simulink model "Model_turn"  (R2024a)
settings: Solver=VariableStepAuto  StartTime=0.0  StopTime=100  MaxStep=0.1  RelTol=1e-3
values from neighbouring files (symbols this model uses):
  c_SMA = 837.36    [params.m]
  Fmax_SMA = 10    [params.m]
  h_SMA = .3    (= 0.3)    [params.m]
  k_gn = m*g/0.01    (= 9810)    [contact3D_params.m]
  k_gt = m*g/0.1    (= 981)    [contact3D_params.m]
  m = 10    [contact3D_params.m]
  m_SMA = 0.0025    [params.m]
  max_SMA_Energy_J = 150    [params.m]
  mu_slide = 0.8    [contact3D_params.m]
  mu_stick = 0.9    [contact3D_params.m]
  n_segs = 10    [params.m]
  PWM_max = 0.35    [params.m]
  R_SMA = .08    (= 0.08)    [params.m]
  r_SMA2limb = 0.009    [params.m]
  swing_angle = swing_angles(i)    [params.m]
  T_amb = 23    [params.m]
  V_0 = 7    [params.m]
  v_gn_max = 0.03    [contact3D_params.m]
  v_gt_max = 0.03    [contact3D_params.m]
  vLimit = 0.01    [contact3D_params.m]
undefined symbols (not defined in the file or in its folder): Newton, Raphson, X, Y, Z
libraries: sm_lib x225, nesl_utility x185, simulink x24, simulink_extras x6
(part 12 of 16)

== system Model_turn/LIMB 1: Back LEFT/Limb 1/Limb_Segment5/Limb_Segment_Torques ==
  In1 : Inport
  In2 : Inport  Port=2
  In3 : Inport  Port=3
  In4 : Inport  Port=4
  Constant{,1..3} (4 alike) : Constant  Value=r_SMA2limb
  Gain{,1..3} (4 alike) : Gain  Gain=1/n_segs
  Product{,1..3} (4 alike) : Product
  Simulink-PS Converter : nesl_utility/Simulink-PS Converter  PhysicalDomain=network_engine_domain  SubClassName=ps_input  LeftPortType=input  RightPortType=output  PseudoPeriodic=off  Frequencies=[]  NoiseDistribution=none  NoiseParameters=[]  Unit=1  AffineConversion=off  FilteringAndDerivatives=provide  SimscapeFilterOrder=1  InputFilterTimeConstant=0.001  UdotUserProvided=0
  Simulink-PS Converter1 : nesl_utility/Simulink-PS Converter  PhysicalDomain=network_engine_domain  SubClassName=ps_input  LeftPortType=input  RightPortType=output  PseudoPeriodic=off  Frequencies=[]  NoiseDistribution=none  NoiseParameters=[]  Unit=1  AffineConversion=off  FilteringAndDerivatives=provide  SimscapeFilterOrder=1  InputFilterTimeConstant=0.001  UdotUserProvided=0
  Sum : Sum  Inputs=+-
  Sum1 : Sum  Inputs=+-
  Torque_X : PMIOPort  Side=Right
  Torque_Y : PMIOPort  Port=2  Side=Right
  wires:
  In3/1 -> Gain2/1
  In1/1 -> Gain/1
  In2/1 -> Gain1/1
  Gain1/1 -> Product1/2
  Gain2/1 -> Product2/2
  Gain/1 -> Product/2
  Product/1 -> Sum/1  "SMA_Torque"
  Product2/1 -> Sum1/1  "SMA_Torque"
  Gain3/1 -> Product3/2
  Constant/1 -> Product/1
  Constant1/1 -> Product1/1
  Product1/1 -> Sum/2  "SMA_Torque"
  In4/1 -> Gain3/1
  Constant3/1 -> Product3/1
  Constant2/1 -> Product2/1
  Sum/1 -> Simulink-PS Converter/1
  Product3/1 -> Sum1/2  "SMA_Torque"
  Sum1/1 -> Simulink-PS Converter1/1
  connections:
  Simulink-PS Converter/RConn1 -- Torque_X/RConn1
  Simulink-PS Converter1/RConn1 -- Torque_Y/RConn1

== system Model_turn/LIMB 1: Back LEFT/Limb 1/Limb_Segment6/Limb_Segment_Torques ==
  In1 : Inport
  In2 : Inport  Port=2
  In3 : Inport  Port=3
  In4 : Inport  Port=4
  Constant{,1..3} (4 alike) : Constant  Value=r_SMA2limb
  Gain{,1..3} (4 alike) : Gain  Gain=1/n_segs
  Product{,1..3} (4 alike) : Product
  Simulink-PS Converter : nesl_utility/Simulink-PS Converter  PhysicalDomain=network_engine_domain  SubClassName=ps_input  LeftPortType=input  RightPortType=output  PseudoPeriodic=off  Frequencies=[]  NoiseDistribution=none  NoiseParameters=[]  Unit=1  AffineConversion=off  FilteringAndDerivatives=provide  SimscapeFilterOrder=1  InputFilterTimeConstant=0.001  UdotUserProvided=0
  Simulink-PS Converter1 : nesl_utility/Simulink-PS Converter  PhysicalDomain=network_engine_domain  SubClassName=ps_input  LeftPortType=input  RightPortType=output  PseudoPeriodic=off  Frequencies=[]  NoiseDistribution=none  NoiseParameters=[]  Unit=1  AffineConversion=off  FilteringAndDerivatives=provide  SimscapeFilterOrder=1  InputFilterTimeConstant=0.001  UdotUserProvided=0
  Sum : Sum  Inputs=+-
  Sum1 : Sum  Inputs=+-
  Torque_X : PMIOPort  Side=Right
  Torque_Y : PMIOPort  Port=2  Side=Right
  wires:
  Sum1/1 -> Simulink-PS Converter1/1
  Product3/1 -> Sum1/2  "SMA_Torque"
  Sum/1 -> Simulink-PS Converter/1
  Constant2/1 -> Product2/1
  Constant3/1 -> Product3/1
  In4/1 -> Gain3/1
  Product1/1 -> Sum/2  "SMA_Torque"
  Constant1/1 -> Product1/1
  Constant/1 -> Product/1
  Gain3/1 -> Product3/2
  Product2/1 -> Sum1/1  "SMA_Torque"
  Product/1 -> Sum/1  "SMA_Torque"
  Gain/1 -> Product/2
  Gain2/1 -> Product2/2
  Gain1/1 -> Product1/2
  In2/1 -> Gain1/1
  In1/1 -> Gain/1
  In3/1 -> Gain2/1
  connections:
  Simulink-PS Converter1/RConn1 -- Torque_Y/RConn1
  Simulink-PS Converter/RConn1 -- Torque_X/RConn1

== system Model_turn/LIMB 1: Back LEFT/Limb 1/Limb_Segment7/Limb_Segment_Torques ==
  In1 : Inport
  In2 : Inport  Port=2
  In3 : Inport  Port=3
  In4 : Inport  Port=4
  Constant{,1..3} (4 alike) : Constant  Value=r_SMA2limb
  Gain{,1..3} (4 alike) : Gain  Gain=1/n_segs
  Product{,1..3} (4 alike) : Product
  Simulink-PS Converter : nesl_utility/Simulink-PS Converter  PhysicalDomain=network_engine_domain  SubClassName=ps_input  LeftPortType=input  RightPortType=output  PseudoPeriodic=off  Frequencies=[]  NoiseDistribution=none  NoiseParameters=[]  Unit=1  AffineConversion=off  FilteringAndDerivatives=provide  SimscapeFilterOrder=1  InputFilterTimeConstant=0.001  UdotUserProvided=0
  Simulink-PS Converter1 : nesl_utility/Simulink-PS Converter  PhysicalDomain=network_engine_domain  SubClassName=ps_input  LeftPortType=input  RightPortType=output  PseudoPeriodic=off  Frequencies=[]  NoiseDistribution=none  NoiseParameters=[]  Unit=1  AffineConversion=off  FilteringAndDerivatives=provide  SimscapeFilterOrder=1  InputFilterTimeConstant=0.001  UdotUserProvided=0
  Sum : Sum  Inputs=+-
  Sum1 : Sum  Inputs=+-
  Torque_X : PMIOPort  Side=Right
  Torque_Y : PMIOPort  Port=2  Side=Right
  wires:
  In3/1 -> Gain2/1
  In1/1 -> Gain/1
  In2/1 -> Gain1/1
  Gain1/1 -> Product1/2
  Gain2/1 -> Product2/2
  Gain/1 -> Product/2
  Product/1 -> Sum/1  "SMA_Torque"
  Product2/1 -> Sum1/1  "SMA_Torque"
  Gain3/1 -> Product3/2
  Constant/1 -> Product/1
  Constant1/1 -> Product1/1
  Product1/1 -> Sum/2  "SMA_Torque"
  In4/1 -> Gain3/1
  Constant3/1 -> Product3/1
  Constant2/1 -> Product2/1
  Sum/1 -> Simulink-PS Converter/1
  Product3/1 -> Sum1/2  "SMA_Torque"
  Sum1/1 -> Simulink-PS Converter1/1
  connections:
  Simulink-PS Converter/RConn1 -- Torque_X/RConn1
  Simulink-PS Converter1/RConn1 -- Torque_Y/RConn1

== system Model_turn/LIMB 1: Back LEFT/Limb 1/Limb_Segment8/Limb_Segment_Torques ==
  In1 : Inport
  In2 : Inport  Port=2
  In3 : Inport  Port=3
  In4 : Inport  Port=4
  Constant{,1..3} (4 alike) : Constant  Value=r_SMA2limb
  Gain{,1..3} (4 alike) : Gain  Gain=1/n_segs
  Product{,1..3} (4 alike) : Product
  Simulink-PS Converter : nesl_utility/Simulink-PS Converter  PhysicalDomain=network_engine_domain  SubClassName=ps_input  LeftPortType=input  RightPortType=output  PseudoPeriodic=off  Frequencies=[]  NoiseDistribution=none  NoiseParameters=[]  Unit=1  AffineConversion=off  FilteringAndDerivatives=provide  SimscapeFilterOrder=1  InputFilterTimeConstant=0.001  UdotUserProvided=0
  Simulink-PS Converter1 : nesl_utility/Simulink-PS Converter  PhysicalDomain=network_engine_domain  SubClassName=ps_input  LeftPortType=input  RightPortType=output  PseudoPeriodic=off  Frequencies=[]  NoiseDistribution=none  NoiseParameters=[]  Unit=1  AffineConversion=off  FilteringAndDerivatives=provide  SimscapeFilterOrder=1  InputFilterTimeConstant=0.001  UdotUserProvided=0
  Sum : Sum  Inputs=+-
  Sum1 : Sum  Inputs=+-
  Torque_X : PMIOPort  Side=Right
  Torque_Y : PMIOPort  Port=2  Side=Right
  wires:
  Sum1/1 -> Simulink-PS Converter1/1
  Product3/1 -> Sum1/2  "SMA_Torque"
  Sum/1 -> Simulink-PS Converter/1
  Constant2/1 -> Product2/1
  Constant3/1 -> Product3/1
  In4/1 -> Gain3/1
  Product1/1 -> Sum/2  "SMA_Torque"
  Constant1/1 -> Product1/1
  Constant/1 -> Product/1
  Gain3/1 -> Product3/2
  Product2/1 -> Sum1/1  "SMA_Torque"
  Product/1 -> Sum/1  "SMA_Torque"
  Gain/1 -> Product/2
  Gain2/1 -> Product2/2
  Gain1/1 -> Product1/2
  In2/1 -> Gain1/1
  In1/1 -> Gain/1
  In3/1 -> Gain2/1
  connections:
  Simulink-PS Converter1/RConn1 -- Torque_Y/RConn1
  Simulink-PS Converter/RConn1 -- Torque_X/RConn1

== system Model_turn/LIMB 1: Back LEFT/Limb 1/Limb_Segment9/Limb_Segment_Torques ==
  In1 : Inport
  In2 : Inport  Port=2
  In3 : Inport  Port=3
  In4 : Inport  Port=4
  Constant{,1..3} (4 alike) : Constant  Value=r_SMA2limb
  Gain{,1..3} (4 alike) : Gain  Gain=1/n_segs
  Product{,1..3} (4 alike) : Product
  Simulink-PS Converter : nesl_utility/Simulink-PS Converter  PhysicalDomain=network_engine_domain  SubClassName=ps_input  LeftPortType=input  RightPortType=output  PseudoPeriodic=off  Frequencies=[]  NoiseDistribution=none  NoiseParameters=[]  Unit=1  AffineConversion=off  FilteringAndDerivatives=provide  SimscapeFilterOrder=1  InputFilterTimeConstant=0.001  UdotUserProvided=0
  Simulink-PS Converter1 : nesl_utility/Simulink-PS Converter  PhysicalDomain=network_engine_domain  SubClassName=ps_input  LeftPortType=input  RightPortType=output  PseudoPeriodic=off  Frequencies=[]  NoiseDistribution=none  NoiseParameters=[]  Unit=1  AffineConversion=off  FilteringAndDerivatives=provide  SimscapeFilterOrder=1  InputFilterTimeConstant=0.001  UdotUserProvided=0
  Sum : Sum  Inputs=+-
  Sum1 : Sum  Inputs=+-
  Torque_X : PMIOPort  Side=Right
  Torque_Y : PMIOPort  Port=2  Side=Right
  wires:
  In3/1 -> Gain2/1
  In1/1 -> Gain/1
  In2/1 -> Gain1/1
  Gain1/1 -> Product1/2
  Gain2/1 -> Product2/2
  Gain/1 -> Product/2
  Product/1 -> Sum/1  "SMA_Torque"
  Product2/1 -> Sum1/1  "SMA_Torque"
  Gain3/1 -> Product3/2
  Constant/1 -> Product/1
  Constant1/1 -> Product1/1
  Product1/1 -> Sum/2  "SMA_Torque"
  In4/1 -> Gain3/1
  Constant3/1 -> Product3/1
  Constant2/1 -> Product2/1
  Sum/1 -> Simulink-PS Converter/1
  Product3/1 -> Sum1/2  "SMA_Torque"
  Sum1/1 -> Simulink-PS Converter1/1
  connections:
  Simulink-PS Converter/RConn1 -- Torque_X/RConn1
  Simulink-PS Converter1/RConn1 -- Torque_Y/RConn1

== system Model_turn/LIMB 1: Back LEFT/Limb 1/Right Ball Contact/3D Contact ==
  RefPt [m m m] : Inport
  nVec [m m m] : Inport  Port=2
  pVec [m m m] : Inport  Port=3
  vVec [m/s m/s m/s] : Inport  Port=4
  Contact! : EnablePort  StatesWhenEnabling=reset
  Friction Switch : Subsystem
  Kinetic Friction Model : Subsystem
  Logical Operator : Logic  Operator=NOT  AllPortsSameDT=off  OutDataTypeStr=boolean
  Static Friction Model : Subsystem
  Sum : Sum
  Sum1 : Sum
  FnVec [N N N] : Outport  OutputWhenDisabled=reset  InitialOutput=[0 0 0]
      settings: AttributesFormatString=when disabled: %<OutputWhenDisabled>
  FtVec [N N N] : Outport  Port=2  OutputWhenDisabled=reset  InitialOutput=[0 0 0]
      settings: AttributesFormatString=when disabled: %<OutputWhenDisabled>
  wires:
  pVec [m m m]/1 -> Static Friction Model/1(pos [m]), Kinetic Friction Model/2(pos [m m m])
  vVec [m/s m/s m/s]/1 -> Kinetic Friction Model/1(vel [m/s m/s m/s]), Static Friction Model/2(vel [m/s m/s m/s])
  Kinetic Friction Model/2(posFP [m m m]) -> Static Friction Model/4(posFP [m])
  Friction Switch/1(Stiction) -> Static Friction Model/Enable, Logical Operator/1
  Logical Operator/1 -> Kinetic Friction Model/Enable
  nVec [m m m]/1 -> Kinetic Friction Model/4(nVec [m m m])
  Kinetic Friction Model/4(Stiction!) -> Friction Switch/2(Stick!)
  Static Friction Model/1(F_n Stick [N N N]) -> Sum1/1
  Kinetic Friction Model/6(F_n Slide [N N N]) -> Sum1/2
  Kinetic Friction Model/5(F_t Slide [N N N]) -> Sum/2
  Static Friction Model/2(F_t Stick [N N N]) -> Sum/1
  Sum1/1 -> FnVec [N N N]/1  "F_nVec"
  Sum/1 -> FtVec [N N N]/1  "F_tVec"
  Static Friction Model/3(Sliding!) -> Friction Switch/1(Slide!)
  RefPt [m m m]/1 -> Kinetic Friction Model/3(RefPt [m m m])
  Kinetic Friction Model/3(nVec FP [m m m]) -> Static Friction Model/5(nVecFP [m m m])
  Kinetic Friction Model/1(RefPtFP [m m m]) -> Static Friction Model/3(RefPtFP [m m m])

== system Model_turn/LIMB 1: Back RIGHT/Limb 1/Limb_Segment/Limb_Segment_Torques ==
  In1 : Inport
  In2 : Inport  Port=2
  In3 : Inport  Port=3
  In4 : Inport  Port=4
  Constant{,1..3} (4 alike) : Constant  Value=r_SMA2limb
  Gain{,1..3} (4 alike) : Gain  Gain=1/n_segs
  Product{,1..3} (4 alike) : Product
  Simulink-PS Converter : nesl_utility/Simulink-PS Converter  PhysicalDomain=network_engine_domain  SubClassName=ps_input  LeftPortType=input  RightPortType=output  PseudoPeriodic=off  Frequencies=[]  NoiseDistribution=none  NoiseParameters=[]  Unit=1  AffineConversion=off  FilteringAndDerivatives=provide  SimscapeFilterOrder=1  InputFilterTimeConstant=0.001  UdotUserProvided=0
  Simulink-PS Converter1 : nesl_utility/Simulink-PS Converter  PhysicalDomain=network_engine_domain  SubClassName=ps_input  LeftPortType=input  RightPortType=output  PseudoPeriodic=off  Frequencies=[]  NoiseDistribution=none  NoiseParameters=[]  Unit=1  AffineConversion=off  FilteringAndDerivatives=provide  SimscapeFilterOrder=1  InputFilterTimeConstant=0.001  UdotUserProvided=0
  Sum : Sum  Inputs=+-
  Sum1 : Sum  Inputs=+-
  Torque_X : PMIOPort  Side=Right
  Torque_Y : PMIOPort  Port=2  Side=Right
  wires:
  Sum1/1 -> Simulink-PS Converter1/1
  Product3/1 -> Sum1/2  "SMA_Torque"
  Sum/1 -> Simulink-PS Converter/1
  Constant2/1 -> Product2/1
  Constant3/1 -> Product3/1
  In4/1 -> Gain3/1
  Product1/1 -> Sum/2  "SMA_Torque"
  Constant1/1 -> Product1/1
  Constant/1 -> Product/1
  Gain3/1 -> Product3/2
  Product2/1 -> Sum1/1  "SMA_Torque"
  Product/1 -> Sum/1  "SMA_Torque"
  Gain/1 -> Product/2
  Gain2/1 -> Product2/2
  Gain1/1 -> Product1/2
  In2/1 -> Gain1/1
  In1/1 -> Gain/1
  In3/1 -> Gain2/1
  connections:
  Simulink-PS Converter1/RConn1 -- Torque_Y/RConn1
  Simulink-PS Converter/RConn1 -- Torque_X/RConn1

== system Model_turn/LIMB 1: Back RIGHT/Limb 1/Limb_Segment1/Limb_Segment_Torques ==
  In1 : Inport
  In2 : Inport  Port=2
  In3 : Inport  Port=3
  In4 : Inport  Port=4
  Constant{,1..3} (4 alike) : Constant  Value=r_SMA2limb
  Gain{,1..3} (4 alike) : Gain  Gain=1/n_segs
  Product{,1..3} (4 alike) : Product
  Simulink-PS Converter : nesl_utility/Simulink-PS Converter  PhysicalDomain=network_engine_domain  SubClassName=ps_input  LeftPortType=input  RightPortType=output  PseudoPeriodic=off  Frequencies=[]  NoiseDistribution=none  NoiseParameters=[]  Unit=1  AffineConversion=off  FilteringAndDerivatives=provide  SimscapeFilterOrder=1  InputFilterTimeConstant=0.001  UdotUserProvided=0
  Simulink-PS Converter1 : nesl_utility/Simulink-PS Converter  PhysicalDomain=network_engine_domain  SubClassName=ps_input  LeftPortType=input  RightPortType=output  PseudoPeriodic=off  Frequencies=[]  NoiseDistribution=none  NoiseParameters=[]  Unit=1  AffineConversion=off  FilteringAndDerivatives=provide  SimscapeFilterOrder=1  InputFilterTimeConstant=0.001  UdotUserProvided=0
  Sum : Sum  Inputs=+-
  Sum1 : Sum  Inputs=+-
  Torque_X : PMIOPort  Side=Right
  Torque_Y : PMIOPort  Port=2  Side=Right
  wires:
  In3/1 -> Gain2/1
  In1/1 -> Gain/1
  In2/1 -> Gain1/1
  Gain1/1 -> Product1/2
  Gain2/1 -> Product2/2
  Gain/1 -> Product/2
  Product/1 -> Sum/1  "SMA_Torque"
  Product2/1 -> Sum1/1  "SMA_Torque"
  Gain3/1 -> Product3/2
  Constant/1 -> Product/1
  Constant1/1 -> Product1/1
  Product1/1 -> Sum/2  "SMA_Torque"
  In4/1 -> Gain3/1
  Constant3/1 -> Product3/1
  Constant2/1 -> Product2/1
  Sum/1 -> Simulink-PS Converter/1
  Product3/1 -> Sum1/2  "SMA_Torque"
  Sum1/1 -> Simulink-PS Converter1/1
  connections:
  Simulink-PS Converter/RConn1 -- Torque_X/RConn1
  Simulink-PS Converter1/RConn1 -- Torque_Y/RConn1

== system Model_turn/LIMB 1: Back RIGHT/Limb 1/Limb_Segment2/Limb_Segment_Torques ==
  In1 : Inport
  In2 : Inport  Port=2
  In3 : Inport  Port=3
  In4 : Inport  Port=4
  Constant{,1..3} (4 alike) : Constant  Value=r_SMA2limb
  Gain{,1..3} (4 alike) : Gain  Gain=1/n_segs
  Product{,1..3} (4 alike) : Product
  Simulink-PS Converter : nesl_utility/Simulink-PS Converter  PhysicalDomain=network_engine_domain  SubClassName=ps_input  LeftPortType=input  RightPortType=output  PseudoPeriodic=off  Frequencies=[]  NoiseDistribution=none  NoiseParameters=[]  Unit=1  AffineConversion=off  FilteringAndDerivatives=provide  SimscapeFilterOrder=1  InputFilterTimeConstant=0.001  UdotUserProvided=0
  Simulink-PS Converter1 : nesl_utility/Simulink-PS Converter  PhysicalDomain=network_engine_domain  SubClassName=ps_input  LeftPortType=input  RightPortType=output  PseudoPeriodic=off  Frequencies=[]  NoiseDistribution=none  NoiseParameters=[]  Unit=1  AffineConversion=off  FilteringAndDerivatives=provide  SimscapeFilterOrder=1  InputFilterTimeConstant=0.001  UdotUserProvided=0
  Sum : Sum  Inputs=+-
  Sum1 : Sum  Inputs=+-
  Torque_X : PMIOPort  Side=Right
  Torque_Y : PMIOPort  Port=2  Side=Right
  wires:
  Sum1/1 -> Simulink-PS Converter1/1
  Product3/1 -> Sum1/2  "SMA_Torque"
  Sum/1 -> Simulink-PS Converter/1
  Constant2/1 -> Product2/1
  Constant3/1 -> Product3/1
  In4/1 -> Gain3/1
  Product1/1 -> Sum/2  "SMA_Torque"
  Constant1/1 -> Product1/1
  Constant/1 -> Product/1
  Gain3/1 -> Product3/2
  Product2/1 -> Sum1/1  "SMA_Torque"
  Product/1 -> Sum/1  "SMA_Torque"
  Gain/1 -> Product/2
  Gain2/1 -> Product2/2
  Gain1/1 -> Product1/2
  In2/1 -> Gain1/1
  In1/1 -> Gain/1
  In3/1 -> Gain2/1
  connections:
  Simulink-PS Converter1/RConn1 -- Torque_Y/RConn1
  Simulink-PS Converter/RConn1 -- Torque_X/RConn1

== system Model_turn/LIMB 1: Back RIGHT/Limb 1/Limb_Segment3/Limb_Segment_Torques ==
  In1 : Inport
  In2 : Inport  Port=2
  In3 : Inport  Port=3
  In4 : Inport  Port=4
  Constant{,1..3} (4 alike) : Constant  Value=r_SMA2limb
  Gain{,1..3} (4 alike) : Gain  Gain=1/n_segs
  Product{,1..3} (4 alike) : Product
  Simulink-PS Converter : nesl_utility/Simulink-PS Converter  PhysicalDomain=network_engine_domain  SubClassName=ps_input  LeftPortType=input  RightPortType=output  PseudoPeriodic=off  Frequencies=[]  NoiseDistribution=none  NoiseParameters=[]  Unit=1  AffineConversion=off  FilteringAndDerivatives=provide  SimscapeFilterOrder=1  InputFilterTimeConstant=0.001  UdotUserProvided=0
  Simulink-PS Converter1 : nesl_utility/Simulink-PS Converter  PhysicalDomain=network_engine_domain  SubClassName=ps_input  LeftPortType=input  RightPortType=output  PseudoPeriodic=off  Frequencies=[]  NoiseDistribution=none  NoiseParameters=[]  Unit=1  AffineConversion=off  FilteringAndDerivatives=provide  SimscapeFilterOrder=1  InputFilterTimeConstant=0.001  UdotUserProvided=0
  Sum : Sum  Inputs=+-
  Sum1 : Sum  Inputs=+-
  Torque_X : PMIOPort  Side=Right
  Torque_Y : PMIOPort  Port=2  Side=Right
  wires:
  In3/1 -> Gain2/1
  In1/1 -> Gain/1
  In2/1 -> Gain1/1
  Gain1/1 -> Product1/2
  Gain2/1 -> Product2/2
  Gain/1 -> Product/2
  Product/1 -> Sum/1  "SMA_Torque"
  Product2/1 -> Sum1/1  "SMA_Torque"
  Gain3/1 -> Product3/2
  Constant/1 -> Product/1
  Constant1/1 -> Product1/1
  Product1/1 -> Sum/2  "SMA_Torque"
  In4/1 -> Gain3/1
  Constant3/1 -> Product3/1
  Constant2/1 -> Product2/1
  Sum/1 -> Simulink-PS Converter/1
  Product3/1 -> Sum1/2  "SMA_Torque"
  Sum1/1 -> Simulink-PS Converter1/1
  connections:
  Simulink-PS Converter/RConn1 -- Torque_X/RConn1
  Simulink-PS Converter1/RConn1 -- Torque_Y/RConn1

== system Model_turn/LIMB 1: Back RIGHT/Limb 1/Limb_Segment4/Limb_Segment_Torques ==
  In1 : Inport
  In2 : Inport  Port=2
  In3 : Inport  Port=3
  In4 : Inport  Port=4
  Constant{,1..3} (4 alike) : Constant  Value=r_SMA2limb
  Gain{,1..3} (4 alike) : Gain  Gain=1/n_segs
  Product{,1..3} (4 alike) : Product
  Simulink-PS Converter : nesl_utility/Simulink-PS Converter  PhysicalDomain=network_engine_domain  SubClassName=ps_input  LeftPortType=input  RightPortType=output  PseudoPeriodic=off  Frequencies=[]  NoiseDistribution=none  NoiseParameters=[]  Unit=1  AffineConversion=off  FilteringAndDerivatives=provide  SimscapeFilterOrder=1  InputFilterTimeConstant=0.001  UdotUserProvided=0
  Simulink-PS Converter1 : nesl_utility/Simulink-PS Converter  PhysicalDomain=network_engine_domain  SubClassName=ps_input  LeftPortType=input  RightPortType=output  PseudoPeriodic=off  Frequencies=[]  NoiseDistribution=none  NoiseParameters=[]  Unit=1  AffineConversion=off  FilteringAndDerivatives=provide  SimscapeFilterOrder=1  InputFilterTimeConstant=0.001  UdotUserProvided=0
  Sum : Sum  Inputs=+-
  Sum1 : Sum  Inputs=+-
  Torque_X : PMIOPort  Side=Right
  Torque_Y : PMIOPort  Port=2  Side=Right
  wires:
  Sum1/1 -> Simulink-PS Converter1/1
  Product3/1 -> Sum1/2  "SMA_Torque"
  Sum/1 -> Simulink-PS Converter/1
  Constant2/1 -> Product2/1
  Constant3/1 -> Product3/1
  In4/1 -> Gain3/1
  Product1/1 -> Sum/2  "SMA_Torque"
  Constant1/1 -> Product1/1
  Constant/1 -> Product/1
  Gain3/1 -> Product3/2
  Product2/1 -> Sum1/1  "SMA_Torque"
  Product/1 -> Sum/1  "SMA_Torque"
  Gain/1 -> Product/2
  Gain2/1 -> Product2/2
  Gain1/1 -> Product1/2
  In2/1 -> Gain1/1
  In1/1 -> Gain/1
  In3/1 -> Gain2/1
  connections:
  Simulink-PS Converter1/RConn1 -- Torque_Y/RConn1
  Simulink-PS Converter/RConn1 -- Torque_X/RConn1

== system Model_turn/LIMB 1: Back RIGHT/Limb 1/Limb_Segment5/Limb_Segment_Torques ==
  In1 : Inport
  In2 : Inport  Port=2
  In3 : Inport  Port=3
  In4 : Inport  Port=4
  Constant{,1..3} (4 alike) : Constant  Value=r_SMA2limb
  Gain{,1..3} (4 alike) : Gain  Gain=1/n_segs
  Product{,1..3} (4 alike) : Product
  Simulink-PS Converter : nesl_utility/Simulink-PS Converter  PhysicalDomain=network_engine_domain  SubClassName=ps_input  LeftPortType=input  RightPortType=output  PseudoPeriodic=off  Frequencies=[]  NoiseDistribution=none  NoiseParameters=[]  Unit=1  AffineConversion=off  FilteringAndDerivatives=provide  SimscapeFilterOrder=1  InputFilterTimeConstant=0.001  UdotUserProvided=0
  Simulink-PS Converter1 : nesl_utility/Simulink-PS Converter  PhysicalDomain=network_engine_domain  SubClassName=ps_input  LeftPortType=input  RightPortType=output  PseudoPeriodic=off  Frequencies=[]  NoiseDistribution=none  NoiseParameters=[]  Unit=1  AffineConversion=off  FilteringAndDerivatives=provide  SimscapeFilterOrder=1  InputFilterTimeConstant=0.001  UdotUserProvided=0
  Sum : Sum  Inputs=+-
  Sum1 : Sum  Inputs=+-
  Torque_X : PMIOPort  Side=Right
  Torque_Y : PMIOPort  Port=2  Side=Right
  wires:
  Sum1/1 -> Simulink-PS Converter1/1
  Product3/1 -> Sum1/2  "SMA_Torque"
  Sum/1 -> Simulink-PS Converter/1
  Constant2/1 -> Product2/1
  Constant3/1 -> Product3/1
  In4/1 -> Gain3/1
  Product1/1 -> Sum/2  "SMA_Torque"
  Constant1/1 -> Product1/1
  Constant/1 -> Product/1
  Gain3/1 -> Product3/2
  Product2/1 -> Sum1/1  "SMA_Torque"
  Product/1 -> Sum/1  "SMA_Torque"
  Gain/1 -> Product/2
  Gain2/1 -> Product2/2
  Gain1/1 -> Product1/2
  In2/1 -> Gain1/1
  In1/1 -> Gain/1
  In3/1 -> Gain2/1
  connections:
  Simulink-PS Converter1/RConn1 -- Torque_Y/RConn1
  Simulink-PS Converter/RConn1 -- Torque_X/RConn1

== system Model_turn/LIMB 1: Back RIGHT/Limb 1/Limb_Segment6/Limb_Segment_Torques ==
  In1 : Inport
  In2 : Inport  Port=2
  In3 : Inport  Port=3
  In4 : Inport  Port=4
  Constant{,1..3} (4 alike) : Constant  Value=r_SMA2limb
  Gain{,1..3} (4 alike) : Gain  Gain=1/n_segs
  Product{,1..3} (4 alike) : Product
  Simulink-PS Converter : nesl_utility/Simulink-PS Converter  PhysicalDomain=network_engine_domain  SubClassName=ps_input  LeftPortType=input  RightPortType=output  PseudoPeriodic=off  Frequencies=[]  NoiseDistribution=none  NoiseParameters=[]  Unit=1  AffineConversion=off  FilteringAndDerivatives=provide  SimscapeFilterOrder=1  InputFilterTimeConstant=0.001  UdotUserProvided=0
  Simulink-PS Converter1 : nesl_utility/Simulink-PS Converter  PhysicalDomain=network_engine_domain  SubClassName=ps_input  LeftPortType=input  RightPortType=output  PseudoPeriodic=off  Frequencies=[]  NoiseDistribution=none  NoiseParameters=[]  Unit=1  AffineConversion=off  FilteringAndDerivatives=provide  SimscapeFilterOrder=1  InputFilterTimeConstant=0.001  UdotUserProvided=0
  Sum : Sum  Inputs=+-
  Sum1 : Sum  Inputs=+-
  Torque_X : PMIOPort  Side=Right
  Torque_Y : PMIOPort  Port=2  Side=Right
  wires:
  In3/1 -> Gain2/1
  In1/1 -> Gain/1
  In2/1 -> Gain1/1
  Gain1/1 -> Product1/2
  Gain2/1 -> Product2/2
  Gain/1 -> Product/2
  Product/1 -> Sum/1  "SMA_Torque"
  Product2/1 -> Sum1/1  "SMA_Torque"
  Gain3/1 -> Product3/2
  Constant/1 -> Product/1
  Constant1/1 -> Product1/1
  Product1/1 -> Sum/2  "SMA_Torque"
  In4/1 -> Gain3/1
  Constant3/1 -> Product3/1
  Constant2/1 -> Product2/1
  Sum/1 -> Simulink-PS Converter/1
  Product3/1 -> Sum1/2  "SMA_Torque"
  Sum1/1 -> Simulink-PS Converter1/1
  connections:
  Simulink-PS Converter/RConn1 -- Torque_X/RConn1
  Simulink-PS Converter1/RConn1 -- Torque_Y/RConn1

== system Model_turn/LIMB 1: Back RIGHT/Limb 1/Limb_Segment7/Limb_Segment_Torques ==
  In1 : Inport
  In2 : Inport  Port=2
  In3 : Inport  Port=3
  In4 : Inport  Port=4
  Constant{,1..3} (4 alike) : Constant  Value=r_SMA2limb
  Gain{,1..3} (4 alike) : Gain  Gain=1/n_segs
  Product{,1..3} (4 alike) : Product
  Simulink-PS Converter : nesl_utility/Simulink-PS Converter  PhysicalDomain=network_engine_domain  SubClassName=ps_input  LeftPortType=input  RightPortType=output  PseudoPeriodic=off  Frequencies=[]  NoiseDistribution=none  NoiseParameters=[]  Unit=1  AffineConversion=off  FilteringAndDerivatives=provide  SimscapeFilterOrder=1  InputFilterTimeConstant=0.001  UdotUserProvided=0
  Simulink-PS Converter1 : nesl_utility/Simulink-PS Converter  PhysicalDomain=network_engine_domain  SubClassName=ps_input  LeftPortType=input  RightPortType=output  PseudoPeriodic=off  Frequencies=[]  NoiseDistribution=none  NoiseParameters=[]  Unit=1  AffineConversion=off  FilteringAndDerivatives=provide  SimscapeFilterOrder=1  InputFilterTimeConstant=0.001  UdotUserProvided=0
  Sum : Sum  Inputs=+-
  Sum1 : Sum  Inputs=+-
  Torque_X : PMIOPort  Side=Right
  Torque_Y : PMIOPort  Port=2  Side=Right
  wires:
  Sum1/1 -> Simulink-PS Converter1/1
  Product3/1 -> Sum1/2  "SMA_Torque"
  Sum/1 -> Simulink-PS Converter/1
  Constant2/1 -> Product2/1
  Constant3/1 -> Product3/1
  In4/1 -> Gain3/1
  Product1/1 -> Sum/2  "SMA_Torque"
  Constant1/1 -> Product1/1
  Constant/1 -> Product/1
  Gain3/1 -> Product3/2
  Product2/1 -> Sum1/1  "SMA_Torque"
  Product/1 -> Sum/1  "SMA_Torque"
  Gain/1 -> Product/2
  Gain2/1 -> Product2/2
  Gain1/1 -> Product1/2
  In2/1 -> Gain1/1
  In1/1 -> Gain/1
  In3/1 -> Gain2/1
  connections:
  Simulink-PS Converter1/RConn1 -- Torque_Y/RConn1
  Simulink-PS Converter/RConn1 -- Torque_X/RConn1

== system Model_turn/LIMB 1: Back RIGHT/Limb 1/Limb_Segment8/Limb_Segment_Torques ==
  In1 : Inport
  In2 : Inport  Port=2
  In3 : Inport  Port=3
  In4 : Inport  Port=4
  Constant{,1..3} (4 alike) : Constant  Value=r_SMA2limb
  Gain{,1..3} (4 alike) : Gain  Gain=1/n_segs
  Product{,1..3} (4 alike) : Product
  Simulink-PS Converter : nesl_utility/Simulink-PS Converter  PhysicalDomain=network_engine_domain  SubClassName=ps_input  LeftPortType=input  RightPortType=output  PseudoPeriodic=off  Frequencies=[]  NoiseDistribution=none  NoiseParameters=[]  Unit=1  AffineConversion=off  FilteringAndDerivatives=provide  SimscapeFilterOrder=1  InputFilterTimeConstant=0.001  UdotUserProvided=0
  Simulink-PS Converter1 : nesl_utility/Simulink-PS Converter  PhysicalDomain=network_engine_domain  SubClassName=ps_input  LeftPortType=input  RightPortType=output  PseudoPeriodic=off  Frequencies=[]  NoiseDistribution=none  NoiseParameters=[]  Unit=1  AffineConversion=off  FilteringAndDerivatives=provide  SimscapeFilterOrder=1  InputFilterTimeConstant=0.001  UdotUserProvided=0
  Sum : Sum  Inputs=+-
  Sum1 : Sum  Inputs=+-
  Torque_X : PMIOPort  Side=Right
  Torque_Y : PMIOPort  Port=2  Side=Right
  wires:
  In3/1 -> Gain2/1
  In1/1 -> Gain/1
  In2/1 -> Gain1/1
  Gain1/1 -> Product1/2
  Gain2/1 -> Product2/2
  Gain/1 -> Product/2
  Product/1 -> Sum/1  "SMA_Torque"
  Product2/1 -> Sum1/1  "SMA_Torque"
  Gain3/1 -> Product3/2
  Constant/1 -> Product/1
  Constant1/1 -> Product1/1
  Product1/1 -> Sum/2  "SMA_Torque"
  In4/1 -> Gain3/1
  Constant3/1 -> Product3/1
  Constant2/1 -> Product2/1
  Sum/1 -> Simulink-PS Converter/1
  Product3/1 -> Sum1/2  "SMA_Torque"
  Sum1/1 -> Simulink-PS Converter1/1
  connections:
  Simulink-PS Converter/RConn1 -- Torque_X/RConn1
  Simulink-PS Converter1/RConn1 -- Torque_Y/RConn1

== system Model_turn/LIMB 1: Back RIGHT/Limb 1/Limb_Segment9/Limb_Segment_Torques ==
  In1 : Inport
  In2 : Inport  Port=2
  In3 : Inport  Port=3
  In4 : Inport  Port=4
  Constant{,1..3} (4 alike) : Constant  Value=r_SMA2limb
  Gain{,1..3} (4 alike) : Gain  Gain=1/n_segs
  Product{,1..3} (4 alike) : Product
  Simulink-PS Converter : nesl_utility/Simulink-PS Converter  PhysicalDomain=network_engine_domain  SubClassName=ps_input  LeftPortType=input  RightPortType=output  PseudoPeriodic=off  Frequencies=[]  NoiseDistribution=none  NoiseParameters=[]  Unit=1  AffineConversion=off  FilteringAndDerivatives=provide  SimscapeFilterOrder=1  InputFilterTimeConstant=0.001  UdotUserProvided=0
  Simulink-PS Converter1 : nesl_utility/Simulink-PS Converter  PhysicalDomain=network_engine_domain  SubClassName=ps_input  LeftPortType=input  RightPortType=output  PseudoPeriodic=off  Frequencies=[]  NoiseDistribution=none  NoiseParameters=[]  Unit=1  AffineConversion=off  FilteringAndDerivatives=provide  SimscapeFilterOrder=1  InputFilterTimeConstant=0.001  UdotUserProvided=0
  Sum : Sum  Inputs=+-
  Sum1 : Sum  Inputs=+-
  Torque_X : PMIOPort  Side=Right
  Torque_Y : PMIOPort  Port=2  Side=Right
  wires:
  Sum1/1 -> Simulink-PS Converter1/1
  Product3/1 -> Sum1/2  "SMA_Torque"
  Sum/1 -> Simulink-PS Converter/1
  Constant2/1 -> Product2/1
  Constant3/1 -> Product3/1
  In4/1 -> Gain3/1
  Product1/1 -> Sum/2  "SMA_Torque"
  Constant1/1 -> Product1/1
  Constant/1 -> Product/1
  Gain3/1 -> Product3/2
  Product2/1 -> Sum1/1  "SMA_Torque"
  Product/1 -> Sum/1  "SMA_Torque"
  Gain/1 -> Product/2
  Gain2/1 -> Product2/2
  Gain1/1 -> Product1/2
  In2/1 -> Gain1/1
  In1/1 -> Gain/1
  In3/1 -> Gain2/1
  connections:
  Simulink-PS Converter1/RConn1 -- Torque_Y/RConn1
  Simulink-PS Converter/RConn1 -- Torque_X/RConn1

== system Model_turn/LIMB 1: Back RIGHT/Limb 1/Right Ball Contact/3D Contact ==
  RefPt [m m m] : Inport
  nVec [m m m] : Inport  Port=2
  pVec [m m m] : Inport  Port=3
  vVec [m/s m/s m/s] : Inport  Port=4
  Contact! : EnablePort  StatesWhenEnabling=reset
  Friction Switch : Subsystem
  Kinetic Friction Model : Subsystem
  Logical Operator : Logic  Operator=NOT  AllPortsSameDT=off  OutDataTypeStr=boolean
  Static Friction Model : Subsystem
  Sum : Sum
  Sum1 : Sum
  FnVec [N N N] : Outport  OutputWhenDisabled=reset  InitialOutput=[0 0 0]
      settings: AttributesFormatString=when disabled: %<OutputWhenDisabled>
  FtVec [N N N] : Outport  Port=2  OutputWhenDisabled=reset  InitialOutput=[0 0 0]
      settings: AttributesFormatString=when disabled: %<OutputWhenDisabled>
  wires:
  pVec [m m m]/1 -> Static Friction Model/1(pos [m]), Kinetic Friction Model/2(pos [m m m])
  vVec [m/s m/s m/s]/1 -> Kinetic Friction Model/1(vel [m/s m/s m/s]), Static Friction Model/2(vel [m/s m/s m/s])
  Kinetic Friction Model/2(posFP [m m m]) -> Static Friction Model/4(posFP [m])
  Friction Switch/1(Stiction) -> Static Friction Model/Enable, Logical Operator/1
  Logical Operator/1 -> Kinetic Friction Model/Enable
  nVec [m m m]/1 -> Kinetic Friction Model/4(nVec [m m m])
  Kinetic Friction Model/4(Stiction!) -> Friction Switch/2(Stick!)
  Static Friction Model/1(F_n Stick [N N N]) -> Sum1/1
  Kinetic Friction Model/6(F_n Slide [N N N]) -> Sum1/2
  Kinetic Friction Model/5(F_t Slide [N N N]) -> Sum/2
  Static Friction Model/2(F_t Stick [N N N]) -> Sum/1
  Sum1/1 -> FnVec [N N N]/1  "F_nVec"
  Sum/1 -> FtVec [N N N]/1  "F_tVec"
  Static Friction Model/3(Sliding!) -> Friction Switch/1(Slide!)
  RefPt [m m m]/1 -> Kinetic Friction Model/3(RefPt [m m m])
  Kinetic Friction Model/3(nVec FP [m m m]) -> Static Friction Model/5(nVecFP [m m m])
  Kinetic Friction Model/1(RefPtFP [m m m]) -> Static Friction Model/3(RefPtFP [m m m])

== system Model_turn/LIMB 1: Center LEFT/Limb 1/Limb_Segment/Limb_Segment_Torques ==
  In1 : Inport
  In2 : Inport  Port=2
  In3 : Inport  Port=3
  In4 : Inport  Port=4
  Constant{,1..3} (4 alike) : Constant  Value=r_SMA2limb
  Gain{,1..3} (4 alike) : Gain  Gain=1/n_segs
  Product{,1..3} (4 alike) : Product
  Simulink-PS Converter : nesl_utility/Simulink-PS Converter  PhysicalDomain=network_engine_domain  SubClassName=ps_input  LeftPortType=input  RightPortType=output  PseudoPeriodic=off  Frequencies=[]  NoiseDistribution=none  NoiseParameters=[]  Unit=1  AffineConversion=off  FilteringAndDerivatives=provide  SimscapeFilterOrder=1  InputFilterTimeConstant=0.001  UdotUserProvided=0
  Simulink-PS Converter1 : nesl_utility/Simulink-PS Converter  PhysicalDomain=network_engine_domain  SubClassName=ps_input  LeftPortType=input  RightPortType=output  PseudoPeriodic=off  Frequencies=[]  NoiseDistribution=none  NoiseParameters=[]  Unit=1  AffineConversion=off  FilteringAndDerivatives=provide  SimscapeFilterOrder=1  InputFilterTimeConstant=0.001  UdotUserProvided=0
  Sum : Sum  Inputs=+-
  Sum1 : Sum  Inputs=+-
  Torque_X : PMIOPort  Side=Right
  Torque_Y : PMIOPort  Port=2  Side=Right
  wires:
  Sum1/1 -> Simulink-PS Converter1/1
  Product3/1 -> Sum1/2  "SMA_Torque"
  Sum/1 -> Simulink-PS Converter/1
  Constant2/1 -> Product2/1
  Constant3/1 -> Product3/1
  In4/1 -> Gain3/1
  Product1/1 -> Sum/2  "SMA_Torque"
  Constant1/1 -> Product1/1
  Constant/1 -> Product/1
  Gain3/1 -> Product3/2
  Product2/1 -> Sum1/1  "SMA_Torque"
  Product/1 -> Sum/1  "SMA_Torque"
  Gain/1 -> Product/2
  Gain2/1 -> Product2/2
  Gain1/1 -> Product1/2
  In2/1 -> Gain1/1
  In1/1 -> Gain/1
  In3/1 -> Gain2/1
  connections:
  Simulink-PS Converter1/RConn1 -- Torque_Y/RConn1
  Simulink-PS Converter/RConn1 -- Torque_X/RConn1

== system Model_turn/LIMB 1: Center LEFT/Limb 1/Limb_Segment1/Limb_Segment_Torques ==
  In1 : Inport
  In2 : Inport  Port=2
  In3 : Inport  Port=3
  In4 : Inport  Port=4
  Constant{,1..3} (4 alike) : Constant  Value=r_SMA2limb
  Gain{,1..3} (4 alike) : Gain  Gain=1/n_segs
  Product{,1..3} (4 alike) : Product
  Simulink-PS Converter : nesl_utility/Simulink-PS Converter  PhysicalDomain=network_engine_domain  SubClassName=ps_input  LeftPortType=input  RightPortType=output  PseudoPeriodic=off  Frequencies=[]  NoiseDistribution=none  NoiseParameters=[]  Unit=1  AffineConversion=off  FilteringAndDerivatives=provide  SimscapeFilterOrder=1  InputFilterTimeConstant=0.001  UdotUserProvided=0
  Simulink-PS Converter1 : nesl_utility/Simulink-PS Converter  PhysicalDomain=network_engine_domain  SubClassName=ps_input  LeftPortType=input  RightPortType=output  PseudoPeriodic=off  Frequencies=[]  NoiseDistribution=none  NoiseParameters=[]  Unit=1  AffineConversion=off  FilteringAndDerivatives=provide  SimscapeFilterOrder=1  InputFilterTimeConstant=0.001  UdotUserProvided=0
  Sum : Sum  Inputs=+-
  Sum1 : Sum  Inputs=+-
  Torque_X : PMIOPort  Side=Right
  Torque_Y : PMIOPort  Port=2  Side=Right
  wires:
  In3/1 -> Gain2/1
  In1/1 -> Gain/1
  In2/1 -> Gain1/1
  Gain1/1 -> Product1/2
  Gain2/1 -> Product2/2
  Gain/1 -> Product/2
  Product/1 -> Sum/1  "SMA_Torque"
  Product2/1 -> Sum1/1  "SMA_Torque"
  Gain3/1 -> Product3/2
  Constant/1 -> Product/1
  Constant1/1 -> Product1/1
  Product1/1 -> Sum/2  "SMA_Torque"
  In4/1 -> Gain3/1
  Constant3/1 -> Product3/1
  Constant2/1 -> Product2/1
  Sum/1 -> Simulink-PS Converter/1
  Product3/1 -> Sum1/2  "SMA_Torque"
  Sum1/1 -> Simulink-PS Converter1/1
  connections:
  Simulink-PS Converter/RConn1 -- Torque_X/RConn1
  Simulink-PS Converter1/RConn1 -- Torque_Y/RConn1

== system Model_turn/LIMB 1: Center LEFT/Limb 1/Limb_Segment2/Limb_Segment_Torques ==
  In1 : Inport
  In2 : Inport  Port=2
  In3 : Inport  Port=3
  In4 : Inport  Port=4
  Constant{,1..3} (4 alike) : Constant  Value=r_SMA2limb
  Gain{,1..3} (4 alike) : Gain  Gain=1/n_segs
  Product{,1..3} (4 alike) : Product
  Simulink-PS Converter : nesl_utility/Simulink-PS Converter  PhysicalDomain=network_engine_domain  SubClassName=ps_input  LeftPortType=input  RightPortType=output  PseudoPeriodic=off  Frequencies=[]  NoiseDistribution=none  NoiseParameters=[]  Unit=1  AffineConversion=off  FilteringAndDerivatives=provide  SimscapeFilterOrder=1  InputFilterTimeConstant=0.001  UdotUserProvided=0
  Simulink-PS Converter1 : nesl_utility/Simulink-PS Converter  PhysicalDomain=network_engine_domain  SubClassName=ps_input  LeftPortType=input  RightPortType=output  PseudoPeriodic=off  Frequencies=[]  NoiseDistribution=none  NoiseParameters=[]  Unit=1  AffineConversion=off  FilteringAndDerivatives=provide  SimscapeFilterOrder=1  InputFilterTimeConstant=0.001  UdotUserProvided=0
  Sum : Sum  Inputs=+-
  Sum1 : Sum  Inputs=+-
  Torque_X : PMIOPort  Side=Right
  Torque_Y : PMIOPort  Port=2  Side=Right
  wires:
  Sum1/1 -> Simulink-PS Converter1/1
  Product3/1 -> Sum1/2  "SMA_Torque"
  Sum/1 -> Simulink-PS Converter/1
  Constant2/1 -> Product2/1
  Constant3/1 -> Product3/1
  In4/1 -> Gain3/1
  Product1/1 -> Sum/2  "SMA_Torque"
  Constant1/1 -> Product1/1
  Constant/1 -> Product/1
  Gain3/1 -> Product3/2
  Product2/1 -> Sum1/1  "SMA_Torque"
  Product/1 -> Sum/1  "SMA_Torque"
  Gain/1 -> Product/2
  Gain2/1 -> Product2/2
  Gain1/1 -> Product1/2
  In2/1 -> Gain1/1
  In1/1 -> Gain/1
  In3/1 -> Gain2/1
  connections:
  Simulink-PS Converter1/RConn1 -- Torque_Y/RConn1
  Simulink-PS Converter/RConn1 -- Torque_X/RConn1

== system Model_turn/LIMB 1: Center LEFT/Limb 1/Limb_Segment3/Limb_Segment_Torques ==
  In1 : Inport
  In2 : Inport  Port=2
  In3 : Inport  Port=3
  In4 : Inport  Port=4
  Constant{,1..3} (4 alike) : Constant  Value=r_SMA2limb
  Gain{,1..3} (4 alike) : Gain  Gain=1/n_segs
  Product{,1..3} (4 alike) : Product
  Simulink-PS Converter : nesl_utility/Simulink-PS Converter  PhysicalDomain=network_engine_domain  SubClassName=ps_input  LeftPortType=input  RightPortType=output  PseudoPeriodic=off  Frequencies=[]  NoiseDistribution=none  NoiseParameters=[]  Unit=1  AffineConversion=off  FilteringAndDerivatives=provide  SimscapeFilterOrder=1  InputFilterTimeConstant=0.001  UdotUserProvided=0
  Simulink-PS Converter1 : nesl_utility/Simulink-PS Converter  PhysicalDomain=network_engine_domain  SubClassName=ps_input  LeftPortType=input  RightPortType=output  PseudoPeriodic=off  Frequencies=[]  NoiseDistribution=none  NoiseParameters=[]  Unit=1  AffineConversion=off  FilteringAndDerivatives=provide  SimscapeFilterOrder=1  InputFilterTimeConstant=0.001  UdotUserProvided=0
  Sum : Sum  Inputs=+-
  Sum1 : Sum  Inputs=+-
  Torque_X : PMIOPort  Side=Right
  Torque_Y : PMIOPort  Port=2  Side=Right
  wires:
  In3/1 -> Gain2/1
  In1/1 -> Gain/1
  In2/1 -> Gain1/1
  Gain1/1 -> Product1/2
  Gain2/1 -> Product2/2
  Gain/1 -> Product/2
  Product/1 -> Sum/1  "SMA_Torque"
  Product2/1 -> Sum1/1  "SMA_Torque"
  Gain3/1 -> Product3/2
  Constant/1 -> Product/1
  Constant1/1 -> Product1/1
  Product1/1 -> Sum/2  "SMA_Torque"
  In4/1 -> Gain3/1
  Constant3/1 -> Product3/1
  Constant2/1 -> Product2/1
  Sum/1 -> Simulink-PS Converter/1
  Product3/1 -> Sum1/2  "SMA_Torque"
  Sum1/1 -> Simulink-PS Converter1/1
  connections:
  Simulink-PS Converter/RConn1 -- Torque_X/RConn1
  Simulink-PS Converter1/RConn1 -- Torque_Y/RConn1

== system Model_turn/LIMB 1: Center LEFT/Limb 1/Limb_Segment4/Limb_Segment_Torques ==
  In1 : Inport
  In2 : Inport  Port=2
  In3 : Inport  Port=3
  In4 : Inport  Port=4
  Constant{,1..3} (4 alike) : Constant  Value=r_SMA2limb
  Gain{,1..3} (4 alike) : Gain  Gain=1/n_segs
  Product{,1..3} (4 alike) : Product
  Simulink-PS Converter : nesl_utility/Simulink-PS Converter  PhysicalDomain=network_engine_domain  SubClassName=ps_input  LeftPortType=input  RightPortType=output  PseudoPeriodic=off  Frequencies=[]  NoiseDistribution=none  NoiseParameters=[]  Unit=1  AffineConversion=off  FilteringAndDerivatives=provide  SimscapeFilterOrder=1  InputFilterTimeConstant=0.001  UdotUserProvided=0
  Simulink-PS Converter1 : nesl_utility/Simulink-PS Converter  PhysicalDomain=network_engine_domain  SubClassName=ps_input  LeftPortType=input  RightPortType=output  PseudoPeriodic=off  Frequencies=[]  NoiseDistribution=none  NoiseParameters=[]  Unit=1  AffineConversion=off  FilteringAndDerivatives=provide  SimscapeFilterOrder=1  InputFilterTimeConstant=0.001  UdotUserProvided=0
  Sum : Sum  Inputs=+-
  Sum1 : Sum  Inputs=+-
  Torque_X : PMIOPort  Side=Right
  Torque_Y : PMIOPort  Port=2  Side=Right
  wires:
  Sum1/1 -> Simulink-PS Converter1/1
  Product3/1 -> Sum1/2  "SMA_Torque"
  Sum/1 -> Simulink-PS Converter/1
  Constant2/1 -> Product2/1
  Constant3/1 -> Product3/1
  In4/1 -> Gain3/1
  Product1/1 -> Sum/2  "SMA_Torque"
  Constant1/1 -> Product1/1
  Constant/1 -> Product/1
  Gain3/1 -> Product3/2
  Product2/1 -> Sum1/1  "SMA_Torque"
  Product/1 -> Sum/1  "SMA_Torque"
  Gain/1 -> Product/2
  Gain2/1 -> Product2/2
  Gain1/1 -> Product1/2
  In2/1 -> Gain1/1
  In1/1 -> Gain/1
  In3/1 -> Gain2/1
  connections:
  Simulink-PS Converter1/RConn1 -- Torque_Y/RConn1
  Simulink-PS Converter/RConn1 -- Torque_X/RConn1

== system Model_turn/LIMB 1: Center LEFT/Limb 1/Limb_Segment5/Limb_Segment_Torques ==
  In1 : Inport
  In2 : Inport  Port=2
  In3 : Inport  Port=3
  In4 : Inport  Port=4
  Constant{,1..3} (4 alike) : Constant  Value=r_SMA2limb
  Gain{,1..3} (4 alike) : Gain  Gain=1/n_segs
  Product{,1..3} (4 alike) : Product
  Simulink-PS Converter : nesl_utility/Simulink-PS Converter  PhysicalDomain=network_engine_domain  SubClassName=ps_input  LeftPortType=input  RightPortType=output  PseudoPeriodic=off  Frequencies=[]  NoiseDistribution=none  NoiseParameters=[]  Unit=1  AffineConversion=off  FilteringAndDerivatives=provide  SimscapeFilterOrder=1  InputFilterTimeConstant=0.001  UdotUserProvided=0
  Simulink-PS Converter1 : nesl_utility/Simulink-PS Converter  PhysicalDomain=network_engine_domain  SubClassName=ps_input  LeftPortType=input  RightPortType=output  PseudoPeriodic=off  Frequencies=[]  NoiseDistribution=none  NoiseParameters=[]  Unit=1  AffineConversion=off  FilteringAndDerivatives=provide  SimscapeFilterOrder=1  InputFilterTimeConstant=0.001  UdotUserProvided=0
  Sum : Sum  Inputs=+-
  Sum1 : Sum  Inputs=+-
  Torque_X : PMIOPort  Side=Right
  Torque_Y : PMIOPort  Port=2  Side=Right
  wires:
  Sum1/1 -> Simulink-PS Converter1/1
  Product3/1 -> Sum1/2  "SMA_Torque"
  Sum/1 -> Simulink-PS Converter/1
  Constant2/1 -> Product2/1
  Constant3/1 -> Product3/1
  In4/1 -> Gain3/1
  Product1/1 -> Sum/2  "SMA_Torque"
  Constant1/1 -> Product1/1
  Constant/1 -> Product/1
  Gain3/1 -> Product3/2
  Product2/1 -> Sum1/1  "SMA_Torque"
  Product/1 -> Sum/1  "SMA_Torque"
  Gain/1 -> Product/2
  Gain2/1 -> Product2/2
  Gain1/1 -> Product1/2
  In2/1 -> Gain1/1
  In1/1 -> Gain/1
  In3/1 -> Gain2/1
  connections:
  Simulink-PS Converter1/RConn1 -- Torque_Y/RConn1
  Simulink-PS Converter/RConn1 -- Torque_X/RConn1

== system Model_turn/LIMB 1: Center LEFT/Limb 1/Limb_Segment6/Limb_Segment_Torques ==
  In1 : Inport
  In2 : Inport  Port=2
  In3 : Inport  Port=3
  In4 : Inport  Port=4
  Constant{,1..3} (4 alike) : Constant  Value=r_SMA2limb
  Gain{,1..3} (4 alike) : Gain  Gain=1/n_segs
  Product{,1..3} (4 alike) : Product
  Simulink-PS Converter : nesl_utility/Simulink-PS Converter  PhysicalDomain=network_engine_domain  SubClassName=ps_input  LeftPortType=input  RightPortType=output  PseudoPeriodic=off  Frequencies=[]  NoiseDistribution=none  NoiseParameters=[]  Unit=1  AffineConversion=off  FilteringAndDerivatives=provide  SimscapeFilterOrder=1  InputFilterTimeConstant=0.001  UdotUserProvided=0
  Simulink-PS Converter1 : nesl_utility/Simulink-PS Converter  PhysicalDomain=network_engine_domain  SubClassName=ps_input  LeftPortType=input  RightPortType=output  PseudoPeriodic=off  Frequencies=[]  NoiseDistribution=none  NoiseParameters=[]  Unit=1  AffineConversion=off  FilteringAndDerivatives=provide  SimscapeFilterOrder=1  InputFilterTimeConstant=0.001  UdotUserProvided=0
  Sum : Sum  Inputs=+-
  Sum1 : Sum  Inputs=+-
  Torque_X : PMIOPort  Side=Right
  Torque_Y : PMIOPort  Port=2  Side=Right
  wires:
  In3/1 -> Gain2/1
  In1/1 -> Gain/1
  In2/1 -> Gain1/1
  Gain1/1 -> Product1/2
  Gain2/1 -> Product2/2
  Gain/1 -> Product/2
  Product/1 -> Sum/1  "SMA_Torque"
  Product2/1 -> Sum1/1  "SMA_Torque"
  Gain3/1 -> Product3/2
  Constant/1 -> Product/1
  Constant1/1 -> Product1/1
  Product1/1 -> Sum/2  "SMA_Torque"
  In4/1 -> Gain3/1
  Constant3/1 -> Product3/1
  Constant2/1 -> Product2/1
  Sum/1 -> Simulink-PS Converter/1
  Product3/1 -> Sum1/2  "SMA_Torque"
  Sum1/1 -> Simulink-PS Converter1/1
  connections:
  Simulink-PS Converter/RConn1 -- Torque_X/RConn1
  Simulink-PS Converter1/RConn1 -- Torque_Y/RConn1

== system Model_turn/LIMB 1: Center LEFT/Limb 1/Limb_Segment7/Limb_Segment_Torques ==
  In1 : Inport
  In2 : Inport  Port=2
  In3 : Inport  Port=3
  In4 : Inport  Port=4
  Constant{,1..3} (4 alike) : Constant  Value=r_SMA2limb
  Gain{,1..3} (4 alike) : Gain  Gain=1/n_segs
  Product{,1..3} (4 alike) : Product
  Simulink-PS Converter : nesl_utility/Simulink-PS Converter  PhysicalDomain=network_engine_domain  SubClassName=ps_input  LeftPortType=input  RightPortType=output  PseudoPeriodic=off  Frequencies=[]  NoiseDistribution=none  NoiseParameters=[]  Unit=1  AffineConversion=off  FilteringAndDerivatives=provide  SimscapeFilterOrder=1  InputFilterTimeConstant=0.001  UdotUserProvided=0
  Simulink-PS Converter1 : nesl_utility/Simulink-PS Converter  PhysicalDomain=network_engine_domain  SubClassName=ps_input  LeftPortType=input  RightPortType=output  PseudoPeriodic=off  Frequencies=[]  NoiseDistribution=none  NoiseParameters=[]  Unit=1  AffineConversion=off  FilteringAndDerivatives=provide  SimscapeFilterOrder=1  InputFilterTimeConstant=0.001  UdotUserProvided=0
  Sum : Sum  Inputs=+-
  Sum1 : Sum  Inputs=+-
  Torque_X : PMIOPort  Side=Right
  Torque_Y : PMIOPort  Port=2  Side=Right
  wires:
  Sum1/1 -> Simulink-PS Converter1/1
  Product3/1 -> Sum1/2  "SMA_Torque"
  Sum/1 -> Simulink-PS Converter/1
  Constant2/1 -> Product2/1
  Constant3/1 -> Product3/1
  In4/1 -> Gain3/1
  Product1/1 -> Sum/2  "SMA_Torque"
  Constant1/1 -> Product1/1
  Constant/1 -> Product/1
  Gain3/1 -> Product3/2
  Product2/1 -> Sum1/1  "SMA_Torque"
  Product/1 -> Sum/1  "SMA_Torque"
  Gain/1 -> Product/2
  Gain2/1 -> Product2/2
  Gain1/1 -> Product1/2
  In2/1 -> Gain1/1
  In1/1 -> Gain/1
  In3/1 -> Gain2/1
  connections:
  Simulink-PS Converter1/RConn1 -- Torque_Y/RConn1
  Simulink-PS Converter/RConn1 -- Torque_X/RConn1

== system Model_turn/LIMB 1: Center LEFT/Limb 1/Limb_Segment8/Limb_Segment_Torques ==
  In1 : Inport
  In2 : Inport  Port=2
  In3 : Inport  Port=3
  In4 : Inport  Port=4
  Constant{,1..3} (4 alike) : Constant  Value=r_SMA2limb
  Gain{,1..3} (4 alike) : Gain  Gain=1/n_segs
  Product{,1..3} (4 alike) : Product
  Simulink-PS Converter : nesl_utility/Simulink-PS Converter  PhysicalDomain=network_engine_domain  SubClassName=ps_input  LeftPortType=input  RightPortType=output  PseudoPeriodic=off  Frequencies=[]  NoiseDistribution=none  NoiseParameters=[]  Unit=1  AffineConversion=off  FilteringAndDerivatives=provide  SimscapeFilterOrder=1  InputFilterTimeConstant=0.001  UdotUserProvided=0
  Simulink-PS Converter1 : nesl_utility/Simulink-PS Converter  PhysicalDomain=network_engine_domain  SubClassName=ps_input  LeftPortType=input  RightPortType=output  PseudoPeriodic=off  Frequencies=[]  NoiseDistribution=none  NoiseParameters=[]  Unit=1  AffineConversion=off  FilteringAndDerivatives=provide  SimscapeFilterOrder=1  InputFilterTimeConstant=0.001  UdotUserProvided=0
  Sum : Sum  Inputs=+-
  Sum1 : Sum  Inputs=+-
  Torque_X : PMIOPort  Side=Right
  Torque_Y : PMIOPort  Port=2  Side=Right
  wires:
  In3/1 -> Gain2/1
  In1/1 -> Gain/1
  In2/1 -> Gain1/1
  Gain1/1 -> Product1/2
  Gain2/1 -> Product2/2
  Gain/1 -> Product/2
  Product/1 -> Sum/1  "SMA_Torque"
  Product2/1 -> Sum1/1  "SMA_Torque"
  Gain3/1 -> Product3/2
  Constant/1 -> Product/1
  Constant1/1 -> Product1/1
  Product1/1 -> Sum/2  "SMA_Torque"
  In4/1 -> Gain3/1
  Constant3/1 -> Product3/1
  Constant2/1 -> Product2/1
  Sum/1 -> Simulink-PS Converter/1
  Product3/1 -> Sum1/2  "SMA_Torque"
  Sum1/1 -> Simulink-PS Converter1/1
  connections:
  Simulink-PS Converter/RConn1 -- Torque_X/RConn1
  Simulink-PS Converter1/RConn1 -- Torque_Y/RConn1
